simulink model "A24_IM_model"  (R2019b)
settings: Solver=ode5  StartTime=0.0  StopTime=1  FixedStep=1e-6  RelTol=1e-3
InitFcn:
  | Rs=1.405; % Stator Resistor (ohm)
  | Rr=1.395; % Rotor Resistor (ohm)
  | Ls=0.178039; % Stator Inductance (H)
  | Lr=0.178039; % Rotor Inductance (H)
  | Lm=0.1722; % Mutual Inductance (H)
  | J=0.0131; % Motor Inertia (Kg.m^2)
  | P=4; % Pole
  | Tl=26.50; % Load Torque (N.m)
  | w=2*pi*50; % w=2*pi*frequency
  | 
  | %%%%%
  | % Ls=Lls+Lm
  | % Lr=Llr+Lm
  | % Nominal power = 4000 (VA)
  | % Voltage (line-line) = 400 (Vrms)
  | % Frequency = 50 (Hz)
  | % 5.4 HP (4 KW)
libraries: powerlib_meascontrol x2
settings Model: Creator=dell  LastModifiedBy=W002220B
settings DataIOCC: ReturnWorkspaceOutputs=off
settings DebuggingCC: ArithmeticOperatorsInVariantConditions=warning
settings SFSimCC: SimUseLocalCustomCode=off  CustomCodeUndefinedFunction=UseInterfaceOnly
settings RTWCC: RTWUseLocalCustomCode=off
settings CodeAppCC: StateflowObjectComments=on
settings SimscapeCC: SimscapeNormalizeSystem=off

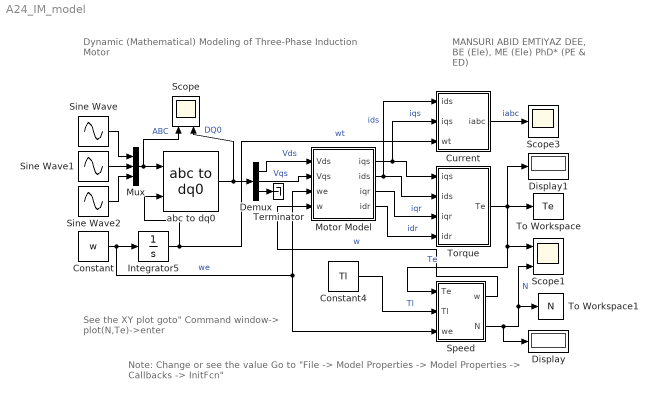
== system A24_IM_model ==
  note: See the XY plot
      | goto" Command window-> plot(N,Te)->enter
  note: Note: Change or see the value
      | Go to "File -> Model Properties -> Model Properties -> Callbacks -> InitFcn"
  note: Dynamic (Mathematical) Modeling of
      | Three-Phase Induction Motor
  note: MANSURI ABID EMTIYAZ
      | DEE, BE (Ele), ME (Ele)
      | PhD* (PE & ED)
  Constant : Constant  Value=w
  Constant4 : Constant  Value=Tl
  Current : Subsystem
  Demux : Demux  Outputs=3
  Display : Display
  Display1 : Display
  Integrator5 : Integrator
  Motor Model : Subsystem
  Mux : Mux  Inputs=3
  Scope : Scope  NumInputPorts=2
  Scope1 : Scope  NumInputPorts=2
  Scope3 : Scope
  Sine Wave : Sin  Amplitude=373.5  Frequency=2*pi*50  SampleTime=0
  Sine Wave1 : Sin  Amplitude=373.5  Frequency=2*pi*50  Phase=-((2*pi)/3)  SampleTime=0
  Sine Wave2 : Sin  Amplitude=373.5  Frequency=2*pi*50  Phase=((2*pi)/3)  SampleTime=0
  Speed : Subsystem
  Terminator : Terminator
  To Workspace : ToWorkspace  VariableName=Te  SampleTime=-1
  To Workspace1 : ToWorkspace  VariableName=N  SampleTime=-1
  Torque : Subsystem
  abc to dq0 : powerlib_meascontrol/Transformations/abc to dq0  Alignment=90 degrees behind phase A axis
      settings: SourceProductName=Simscape Electrical
  wires:
  Sine Wave1/1 -> Mux/2
  Sine Wave/1 -> Mux/1
  Sine Wave2/1 -> Mux/3
  Constant/1 -> Speed/3(we), Motor Model/3(we), Integrator5/1  "we"
  abc to dq0/1 -> Demux/1, Scope/2  "DQ0"
  Integrator5/1 -> Current/3(wt), abc to dq0/2  "wt"
  Constant4/1 -> Speed/2(Tl)  "Tl"
  Demux/1 -> Motor Model/1(Vds)  "Vds"
  Demux/2 -> Motor Model/2(Vqs)  "Vqs"
  Demux/3 -> Terminator/1
  Torque/1(Te) -> To Workspace/1, Speed/1(Te), Scope1/1, Display1/1  "Te"
  Speed/2(N) -> Scope1/2, To Workspace1/1, Display/1  "N"
  Mux/1 -> Scope/1, abc to dq0/1  "ABC"
  Motor Model/1(iqs) -> Torque/1(iqs), Current/2(iqs)  "iqs"
  Motor Model/2(ids) -> Torque/2(ids), Current/1(ids)  "ids"
  Current/1(iabc) -> Scope3/1  "iabc"
  Motor Model/3(iqr) -> Torque/3(iqr)  "iqr"
  Motor Model/4(idr) -> Torque/4(idr)  "idr"
  Speed/1(w) -> Motor Model/4(w)  "w"

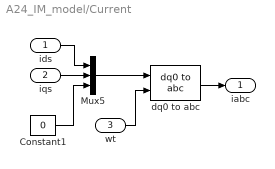
== system A24_IM_model/Current ==
  ids : Inport
  iqs : Inport  Port=2
  wt : Inport  Port=3
  Constant1 : Constant  Value=0
  Mux5 : Mux  Inputs=3
  dq0 to abc : powerlib_meascontrol/Transformations/dq0 to abc  Alignment=90 degrees behind phase A axis
      settings: SourceProductName=Simscape Electrical
  iabc : Outport
  wires:
  dq0 to abc/1 -> iabc/1
  wt/1 -> dq0 to abc/2
  Constant1/1 -> Mux5/3
  iqs/1 -> Mux5/2
  Mux5/1 -> dq0 to abc/1
  ids/1 -> Mux5/1

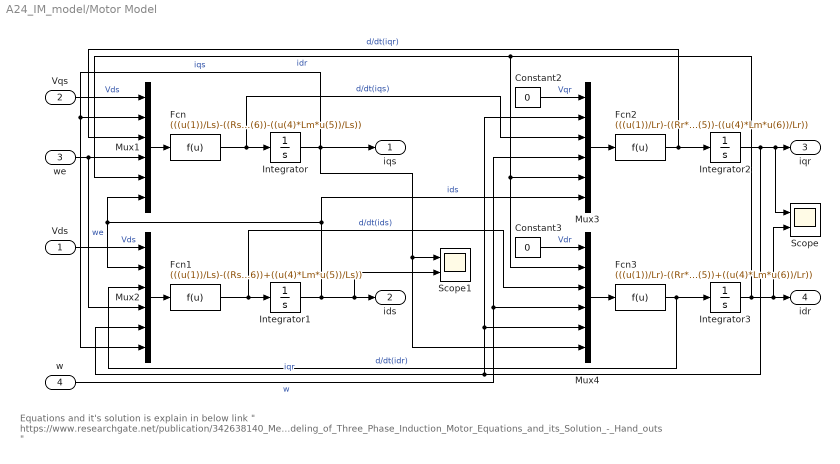
== system A24_IM_model/Motor Model ==
  note: Equations and it's solution is explain in below link
      | " https://www.researchgate.net/publication/342638140_Method-1_Mathematical_Modeling_of_Three_Phase_Induction_Motor_Equations_and_its_Solution_-_Hand_outs "
  Vds : Inport
  Vqs : Inport  Port=2
  we : Inport  Port=3
  w : Inport  Port=4
  Constant2 : Constant  Value=0
  Constant3 : Constant  Value=0
  Fcn : Fcn  Expr=(((u(1))/Ls)-((Rs*u(2))/Ls)-((u(3)*Lm)/Ls)-(u(4)*u(6))-((u(4)*Lm*u(5))/Ls))
  Fcn1 : Fcn  Expr=(((u(1))/Ls)-((Rs*u(2))/Ls)-((u(3)*Lm)/Ls)+(u(4)*u(6))+((u(4)*Lm*u(5))/Ls))
  Fcn2 : Fcn  Expr=(((u(1))/Lr)-((Rr*u(2))/Lr)-((u(3)*Lm)/Lr)-(u(4)*u(5))-((u(4)*Lm*u(6))/Lr))
  Fcn3 : Fcn  Expr=(((u(1))/Lr)-((Rr*u(2))/Lr)-((u(3)*Lm)/Lr)+(u(4)*u(5))+((u(4)*Lm*u(6))/Lr))
  Integrator{,1..3} (4 alike) : Integrator
  Mux{1..4} (4 alike) : Mux  Inputs=6
  Scope : Scope  NumInputPorts=2
  Scope1 : Scope  NumInputPorts=2
  iqs : Outport
  ids : Outport  Port=2
  iqr : Outport  Port=3
  idr : Outport  Port=4
  wires:
  Mux4/1 -> Fcn3/1
  Integrator1/1 -> Scope1/2, ids/1, Mux3/6, Mux1/6, Mux2/2  "ids"
  Constant2/1 -> Mux3/1  "Vqr"
  Mux3/1 -> Fcn2/1
  Mux1/1 -> Fcn/1
  w/1 -> Mux4/4, Mux3/4  "w"
  Fcn1/1 -> Mux4/3, Integrator1/1  "d/dt(ids)"
  Mux2/1 -> Fcn1/1
  Fcn2/1 -> Mux1/3, Integrator2/1  "d/dt(iqr)"
  Constant3/1 -> Mux4/1  "Vdr"
  Fcn3/1 -> Mux2/3, Integrator3/1  "d/dt(idr)"
  Integrator/1 -> Scope1/1, Mux4/6, iqs/1, Mux1/2, Mux2/6  "iqs"
  Fcn/1 -> Mux3/3, Integrator/1  "d/dt(iqs)"
  Vds/1 -> Mux2/1  "Vds"
  we/1 -> Mux2/4, Mux1/4  "we"
  Integrator2/1 -> Scope/1, iqr/1, Mux2/5, Mux4/5, Mux3/2  "iqr"
  Integrator3/1 -> Scope/2, idr/1, Mux1/5, Mux4/2, Mux3/5  "idr"
  Vqs/1 -> Mux1/1  "Vds"

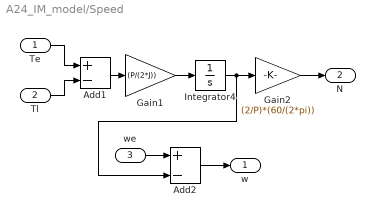
== system A24_IM_model/Speed ==
  Te : Inport
  Tl : Inport  Port=2
  we : Inport  Port=3
  Add1 : Sum  Inputs=+-
  Add2 : Sum  Inputs=+-
  Gain1 : Gain  Gain=(P/(2*J))
  Gain2 : Gain  Gain=(2/P)*(60/(2*pi))
  Integrator4 : Integrator
  w : Outport
  N : Outport  Port=2
  wires:
  Gain1/1 -> Integrator4/1
  Tl/1 -> Add1/2
  Add1/1 -> Gain1/1
  Te/1 -> Add1/1
  Integrator4/1 -> Add2/2, Gain2/1
  we/1 -> Add2/1
  Add2/1 -> w/1
  Gain2/1 -> N/1

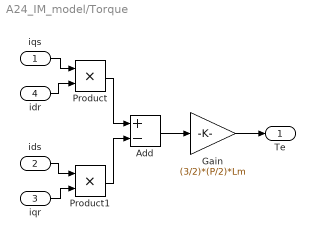
== system A24_IM_model/Torque ==
  iqs : Inport
  ids : Inport  Port=2
  iqr : Inport  Port=3
  idr : Inport  Port=4
  Add : Sum  Inputs=+-
  Gain : Gain  Gain=(3/2)*(P/2)*Lm
  Product : Product
  Product1 : Product
  Te : Outport
  wires:
  Product1/1 -> Add/2
  idr/1 -> Product/2
  Add/1 -> Gain/1
  Product/1 -> Add/1
  iqr/1 -> Product1/2
  Gain/1 -> Te/1
  iqs/1 -> Product/1
  ids/1 -> Product1/1
